simulink model "IPMSM_FOC_FFB"  (R2020b)
settings: Solver=FixedStepDiscrete  StartTime=0.0  StopTime=20  FixedStep=Ts  RelTol=1e-3  EnableMultiTasking=on
InitFcn:
  | Ts=50e-6;     % Simulation time step
  | kp = 100;   % Proportional gain
  | ki =10;   % Integral gain
  | fsw = 2e3;     % Switching frequency
  | Vdc = 400      % Inverter DC supply voltage
  | Rs = 0.1      % Stator resistance
  | Ld = 1e-3    % Inductance (d axis)
  | Lq = 1e-3    % Inductance (q axis)
  | PM = 0.28         % Flux linkage
  | N = 1                % Pole pairs
undefined symbols (not defined in the file): DiscIntNeverNeededParam
libraries: powerlib x7, powerlib_meascontrol x6, eeGeneralControl x2, mcbcontrolslib x1
Description:
  | Copyright 2008-2019 The MathWorks, Inc.
settings Model: SimulationMode=external  ExtModeEnableFloating=off  Creator=MathWorks  LastModifiedBy=Research
settings SolverCC: ConcurrentTasks=on  PositivePriorityOrder=on  AutoInsertRateTranBlk=on
settings DataIOCC: LimitDataPoints=on  SaveFormat=Array  SignalLoggingSaveFormat=ModelDataLogs  SaveOutput=off  SignalLogging=off  SaveTime=off  ReturnWorkspaceOutputs=off  SignalLoggingName=sigsOut
settings OptimizationCC: BlockReduction=off  OptimizeBlockIOStorage=off  ExpressionDepthLimit=2147483647  InitFltsAndDblsToZero=on
settings DebuggingCC: UnderspecifiedInitializationDetection=Classic  MergeDetectMultiDrivingBlocksExec=none  CheckExecutionContextPreStartOutputMsg=on  SignalResolutionControl=TryResolveAllWithWarning  TasksWithSamePriorityMsg=none  FcnCallInpInsideContextMsg=warning  AllowSymbolicDim=off  StateNameClashWarn=warning  SFUnexpectedBacktrackingDiag=warning  SFNoUnconditionalDefaultTransitionDiag=warning  SFExecutionAtInitializationDiag=none  ArithmeticOperatorsInVariantConditions=warning
settings HardwareCC: ProdBitPerLong=64  ProdLongLongMode=on  ProdHWDeviceType=Intel->x86-64 (Linux 64)  TargetBitPerPointer=64  TargetBitPerSizeT=64  TargetBitPerPtrDiffT=64  TargetLongLongMode=on  TargetIntDivRoundTo=Zero  TargetEndianess=LittleEndian  TargetWordSize=64  TargetHWDeviceType=MATLAB Host
settings ModelReferenceCC: PropagateSignalLabelsOutOfModel=off
settings SFSimCC: SimUseLocalCustomCode=off  CustomCodeUndefinedFunction=UseInterfaceOnly
settings RTWCC: Description=Simulink Real-Time  SystemTargetFile=slrealtime.tlc  TemplateMakefile=slrealtime_default_tmf  RTWUseLocalCustomCode=off  Toolchain=Simulink Real-Time Toolchain  BuildConfiguration=Faster Runs  CodeExecutionProfiling=on  TargetLang=C++
settings CodeAppCC: StateflowObjectComments=on
settings ConfigComp: CovMetricSettings=dw  CovSaveCumulativeToWorkspaceVar=on  CovSaveSingleToWorkspaceVar=on  CovExternalEMLEnable=off  CovSFcnEnable=off
settings SimscapeCC: SimscapeNormalizeSystem=off

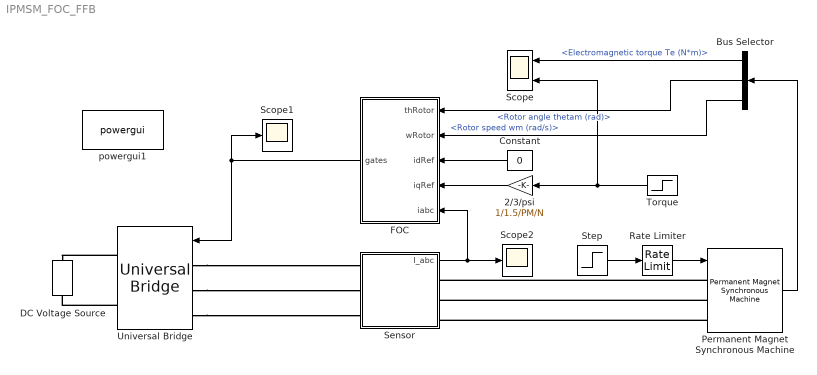
== system IPMSM_FOC_FFB ==
  2/3/psi : Gain  Gain=1/1.5/PM/N  SaturateOnIntegerOverflow=on  OutDataTypeStr=Inherit: Same as input  ParamDataTypeStr=Inherit: Same as input
  Bus Selector : BusSelector  OutputSignals=Electromagnetic torque Te (N*m),Rotor angle thetam (rad),Rotor speed wm (rad/s)
  Constant : Constant  Value=0
  DC Voltage Source : powerlib/Electrical Sources/DC Voltage Source  Amplitude=Vdc  Measurements=None
  FOC : Subsystem
  Permanent Magnet Synchronous Machine : powerlib/Machines/Permanent Magnet Synchronous Machine  NbPhases=3  FluxDistribution=Sinusoidal  RotorType=Salient-pole  MechanicalLoad=Speed w  PresetModel=No  ShowDetailedParameters=on  MeasurementBus=off  Resistance=Rs  Inductance=8.5e-3  dqInductances=[Ld Lq]  La=0.000395  MachineConstant=Flux linkage established by magnets (V.s)  Flux=PM  VoltageCst=32.6484  TorqueCst=0.27  Flat=120  Mechanical=[0.0027 0.0004924 1 0]  PolePairs=N  InitialConditions=[0,0, 0,0]  InitialConditions5ph=[0 0 0 0 0 0]  RefAngle=Aligned with phase A axis (original Park)  IterativeDiscreteModel=Trapezoidal non iterative  TsBlock=-1  TsPowergui=0
  Rate Limiter : RateLimiter  RisingSlewLimit=100/60*2*pi  SampleTimeMode=inherited
  Scope : Scope  NumInputPorts=2
  Scope1 : Scope
  Scope2 : Scope
  Sensor : Subsystem
  Step : Step  Time=0  After=1000/60*2*pi  SampleTime=Ts
  Torque : Step  Time=0.3  After=300
  Universal Bridge : powerlib/Power Electronics/Universal Bridge  Arms=3  SnubberResistance=5000  SnubberCapacitance=inf  Device=Ideal Switches  Ron=1e-4  Lon=0  ForwardVoltages="[  0  0  ]"  ForwardVoltage=0  GTOparameters=[ 10e-6 , 20e-6 ]  IGBTparameters=[ 1e-6 , 2e-6 ]  Measurements=None  Measurements_2=None  converterType=Rectifier
  powergui1 : powerlib/powergui  Priority=1  SimulationMode=Discrete  SampleTime=Ts  frequency=60  Iterations=50  frequencyindice=0  Pbase=100e6  ErrMax=1e-4  UnitsV=kV  UnitsW=MW  buscounter=0  FunctionMessages=off  echomessages=off  EnableUseOfTLC=off  CurrentSourceSwitches=off  DisableSnubberDevices=off  DisableRonSwitches=off  DisableVfSwitches=off  DisplayEquations=off  AutomaticDiscreteSolvers=off  SolverType=Tustin  Interpol=off  ExternalGateDelay=off  methode=off  Ts=100  x0status=blocks  SPID=on  SwTol=0  HookPort=off  NonlinearTolerance=1e-4  nMaxIteration=100  ContinueOnMaxIteration=off  RestoreLinks=warning  ResistiveCurrentMeasurement=off  Frange=[0:2:500]  Ylog=off  Xlog=on  ShowGrid=off  save=off  variable=ZData  structure=0  ZoomFFT=off  StartTime=0.0  cycles=1  DisplayStyle=1  fundamental=60  FreqAxis=off  MaxFrequency=1000  frequencyindicesteady=1  RmsSteady=1  display=off
  wires:
  Permanent Magnet Synchronous Machine/1 -> Bus Selector/1
  Rate Limiter/1 -> Permanent Magnet Synchronous Machine/1
  FOC/1(gates) -> Universal Bridge/1, Scope1/1
  Bus Selector/1 -> Scope/1  "<Electromagnetic torque Te (N*m)>"
  Torque/1 -> 2/3/psi/1, Scope/2
  Sensor/1(I_abc) -> Scope2/1, FOC/5(iabc)
  Constant/1 -> FOC/3(idRef)
  Bus Selector/2 -> FOC/1(thRotor)  "<Rotor angle thetam (rad)>"
  Bus Selector/3 -> FOC/2(wRotor)  "<Rotor speed wm (rad/s)>"
  2/3/psi/1 -> FOC/4(iqRef)
  Step/1 -> Rate Limiter/1
  connections:
  Universal Bridge/RConn2 -- DC Voltage Source/LConn1
  Universal Bridge/LConn1 -- Sensor/LConn1
  Universal Bridge/LConn2 -- Sensor/LConn2
  Permanent Magnet Synchronous Machine/LConn1 -- Sensor/RConn1
  Permanent Magnet Synchronous Machine/LConn2 -- Sensor/RConn2
  Permanent Magnet Synchronous Machine/LConn3 -- Sensor/RConn3
  Universal Bridge/RConn1 -- DC Voltage Source/RConn1
  Universal Bridge/LConn3 -- Sensor/LConn3

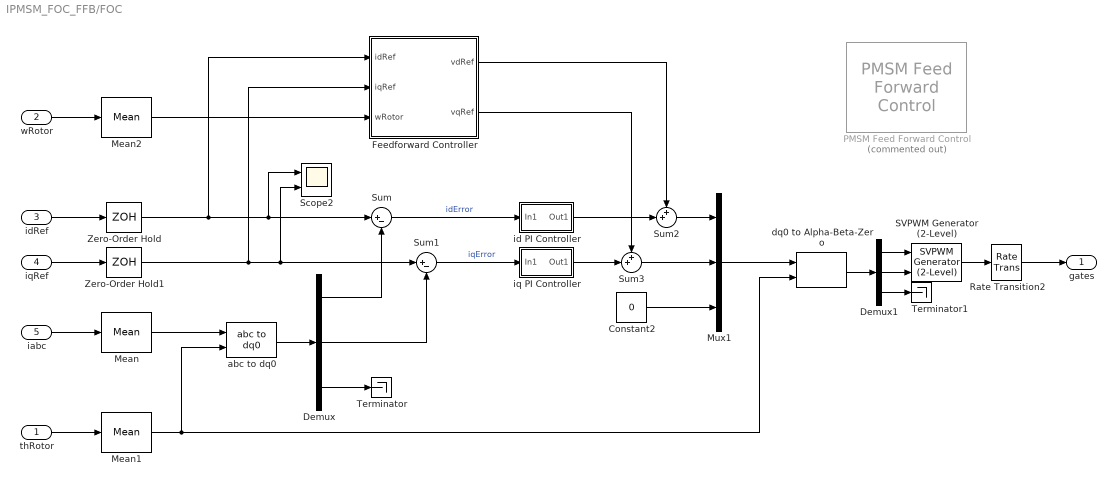
== system IPMSM_FOC_FFB/FOC ==
  thRotor : Inport
  wRotor : Inport  Port=2
  idRef : Inport  Port=3
  iqRef : Inport  Port=4
  iabc : Inport  Port=5
  Constant2 : Constant  Value=0  SampleTime=-1
  Demux : Demux  Outputs=3
  Demux1 : Demux  Outputs=3
  Feedforward Controller : Subsystem
  Mean : powerlib_meascontrol/Measurements/Mean  Freq=fsw  Vinit=0  Ts=Ts
  Mean1 : powerlib_meascontrol/Measurements/Mean  Freq=fsw  Vinit=0  Ts=Ts
  Mean2 : powerlib_meascontrol/Measurements/Mean  Freq=fsw  Vinit=0  Ts=Ts
  Mux1 : Mux  Inputs=3
  PMSM Feed Forward Control : mcbcontrolslib/PMSM Feed Forward Control  Commented=on  polePairs=N  Ld=Ld  Lq=Lq  FluxPM=PM  V_dc=Vdc/sqrt(3)  Units=SI Units  V_base=24/sqrt(3)  I_base=19.3  N_base=4107
      settings: SourceProductBaseCode=MT
  Rate Transition2 : RateTransition
  SVPWM Generator (2-Level) : powerlib_meascontrol/Pulse & Signal Generators/SVPWM Generator (2-Level)  InputType=alpha-beta components  SwitchingPattern=Pattern #1  Fc=fsw  ParUref=[0.8 -30 50]  Ts=Ts
      settings: SourceProductBaseCode=PS
  Scope2 : Scope  NumInputPorts=2
  Sum : Sum  Inputs=|+-
  Sum1 : Sum  Inputs=|+-
  Sum2 : Sum  Inputs=++|
  Sum3 : Sum  Inputs=++|
  Terminator : Terminator
  Terminator1 : Terminator
  Zero-Order Hold : ZeroOrderHold  SampleTime=-1
  Zero-Order Hold1 : ZeroOrderHold  SampleTime=-1
  abc to dq0 : powerlib_meascontrol/Transformations/abc to dq0  Alignment=Aligned with phase A axis
  dq0 to Alpha-Beta-Zero : powerlib_meascontrol/Transformations/dq0 to Alpha-Beta-Zero  Alignment=Aligned with phase A axis
      settings: SourceProductBaseCode=PS
  id PI Controller : Subsystem
  iq PI Controller : Subsystem
  gates : Outport  VectorParamsAs1DForOutWhenUnconnected=off
  wires:
  Demux/3 -> Terminator/1
  iq PI Controller/1(Out1) -> Sum3/2
  Zero-Order Hold/1 -> Feedforward Controller/1(idRef), Scope2/1, Sum/1
  Demux1/1 -> SVPWM Generator (2-Level)/1
  Sum/1 -> id PI Controller/1(In1)  "idError"
  abc to dq0/1 -> Demux/1
  Zero-Order Hold1/1 -> Feedforward Controller/2(iqRef), Sum1/1, Scope2/2
  Rate Transition2/1 -> gates/1
  wRotor/1 -> Mean2/1
  Mean1/1 -> abc to dq0/2, dq0 to Alpha-Beta-Zero/2
  Mean2/1 -> Feedforward Controller/3(wRotor)
  Mean/1 -> abc to dq0/1
  thRotor/1 -> Mean1/1
  Mux1/1 -> dq0 to Alpha-Beta-Zero/1
  Demux1/3 -> Terminator1/1
  iabc/1 -> Mean/1
  Sum1/1 -> iq PI Controller/1(In1)  "iqError"
  Demux/2 -> Sum1/2
  Sum3/1 -> Mux1/2
  Sum2/1 -> Mux1/1
  id PI Controller/1(Out1) -> Sum2/2
  SVPWM Generator (2-Level)/1 -> Rate Transition2/1
  Demux1/2 -> SVPWM Generator (2-Level)/2
  dq0 to Alpha-Beta-Zero/1 -> Demux1/1
  Demux/1 -> Sum/2
  Constant2/1 -> Mux1/3
  Feedforward Controller/1(vdRef) -> Sum2/1
  Feedforward Controller/2(vqRef) -> Sum3/1
  idRef/1 -> Zero-Order Hold/1
  iqRef/1 -> Zero-Order Hold1/1

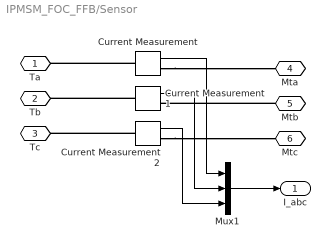
== system IPMSM_FOC_FFB/Sensor ==
  Current Measurement : powerlib/Measurements/Current Measurement  PhasorSimulation=off  OutputType=Complex  PSBequivalent=0
  Current Measurement1 : powerlib/Measurements/Current Measurement  PhasorSimulation=off  OutputType=Complex  PSBequivalent=0
  Current Measurement2 : powerlib/Measurements/Current Measurement  PhasorSimulation=off  OutputType=Complex  PSBequivalent=0
  Mux1 : Mux  Inputs=3
  Ta : PMIOPort  Side=Left
  Tb : PMIOPort  Port=2  Side=Left
  Tc : PMIOPort  Port=3  Side=Left
  Mta : PMIOPort  Port=4  Side=Right
  Mtb : PMIOPort  Port=5  Side=Right
  Mtc : PMIOPort  Port=6  Side=Right
  I_abc : Outport  VectorParamsAs1DForOutWhenUnconnected=off
  wires:
  Current Measurement1/1 -> Mux1/2
  Current Measurement/1 -> Mux1/1
  Current Measurement2/1 -> Mux1/3
  Mux1/1 -> I_abc/1
  connections:
  Mtb/RConn1 -- Current Measurement1/RConn1
  Current Measurement1/LConn1 -- Tb/RConn1
  Current Measurement/RConn1 -- Mta/RConn1
  Current Measurement/LConn1 -- Ta/RConn1
  Current Measurement2/LConn1 -- Tc/RConn1
  Current Measurement2/RConn1 -- Mtc/RConn1

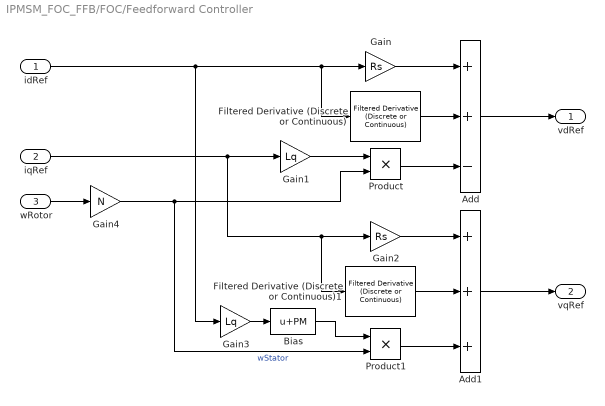
== system IPMSM_FOC_FFB/FOC/Feedforward Controller ==
  idRef : Inport
  iqRef : Inport  Port=2
  wRotor : Inport  Port=3
  Add : Sum  Inputs=++-
  Add1 : Sum  Inputs=+++
  Bias : Bias  Bias=PM  SaturateOnIntegerOverflow=on
  Filtered Derivative (Discrete or Continuous) : eeGeneralControl/Filtered Derivative (Discrete or Continuous)  K=Ld  T=1e-3  B=inf  A=-inf  minRatio=10  init_option=Specify as parameter  x0=0  Ts=-1
      settings: SourceProductBaseCode=PS
  Filtered Derivative (Discrete or Continuous)1 : eeGeneralControl/Filtered Derivative (Discrete or Continuous)  K=Lq  T=1e-3  B=inf  A=-inf  minRatio=10  init_option=Specify as parameter  x0=0  Ts=-1
      settings: SourceProductBaseCode=PS
  Gain : Gain  Gain=Rs
  Gain1 : Gain  Gain=Lq
  Gain2 : Gain  Gain=Rs
  Gain3 : Gain  Gain=Lq
  Gain4 : Gain  Gain=N
  Product : Product
  Product1 : Product
  vdRef : Outport
  vqRef : Outport  Port=2
  wires:
  wRotor/1 -> Gain4/1
  Add/1 -> vdRef/1
  Gain4/1 -> Product/2, Product1/2  "wStator"
  Gain/1 -> Add/1
  idRef/1 -> Gain3/1, Filtered Derivative (Discrete or Continuous)/1, Gain/1
  Gain1/1 -> Product/1
  Product1/1 -> Add1/3
  Gain2/1 -> Add1/1
  Filtered Derivative (Discrete or Continuous)/1 -> Add/2
  iqRef/1 -> Gain2/1, Filtered Derivative (Discrete or Continuous)1/1, Gain1/1
  Filtered Derivative (Discrete or Continuous)1/1 -> Add1/2
  Bias/1 -> Product1/1
  Product/1 -> Add/3
  Gain3/1 -> Bias/1
  Add1/1 -> vqRef/1

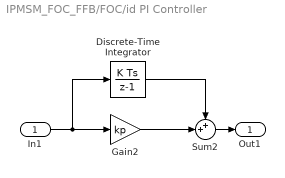
== system IPMSM_FOC_FFB/FOC/id PI Controller ==
  In1 : Inport
  Discrete-Time Integrator : DiscreteIntegrator  gainval=ki  SampleTime=-1  LimitOutput=on  UpperSaturationLimit=1  LowerSaturationLimit=-1  ICPrevOutput=DiscIntNeverNeededParam  ICPrevScaledInput=DiscIntNeverNeededParam
  Gain2 : Gain  Gain=kp  SaturateOnIntegerOverflow=on  OutDataTypeStr=Inherit: Same as input  ParamDataTypeStr=Inherit: Same as input
  Sum2 : Sum  Inputs=++|
  Out1 : Outport  VectorParamsAs1DForOutWhenUnconnected=off
  wires:
  Gain2/1 -> Sum2/2
  In1/1 -> Discrete-Time Integrator/1, Gain2/1
  Sum2/1 -> Out1/1
  Discrete-Time Integrator/1 -> Sum2/1

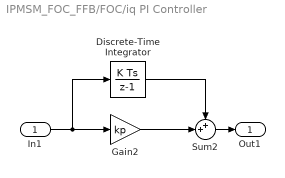
== system IPMSM_FOC_FFB/FOC/iq PI Controller ==
  In1 : Inport
  Discrete-Time Integrator : DiscreteIntegrator  gainval=ki  SampleTime=-1  LimitOutput=on  UpperSaturationLimit=1  LowerSaturationLimit=-1  ICPrevOutput=DiscIntNeverNeededParam  ICPrevScaledInput=DiscIntNeverNeededParam
  Gain2 : Gain  Gain=kp  SaturateOnIntegerOverflow=on  OutDataTypeStr=Inherit: Same as input  ParamDataTypeStr=Inherit: Same as input
  Sum2 : Sum  Inputs=++|
  Out1 : Outport  VectorParamsAs1DForOutWhenUnconnected=off
  wires:
  Gain2/1 -> Sum2/2
  In1/1 -> Discrete-Time Integrator/1, Gain2/1
  Sum2/1 -> Out1/1
  Discrete-Time Integrator/1 -> Sum2/1
